simulink model "W03_P1"  (R2024b)
settings: Solver=ode4  StartTime=0  StopTime=T_final  FixedStep=h  RelTol=1e-3
undefined symbols (not defined in the file or in its folder): beta_c, mp, rp, V_c, x0
settings Model: Creator=admin  LastModifiedBy=admin
settings DataIOCC: ReturnWorkspaceOutputs=off

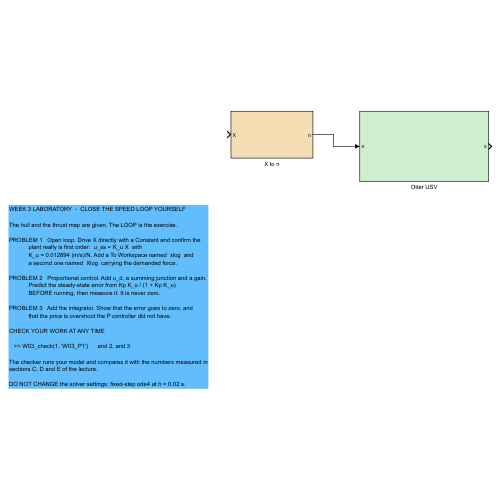
[thumbnail: Simulink's stored preview of the top-level diagram]
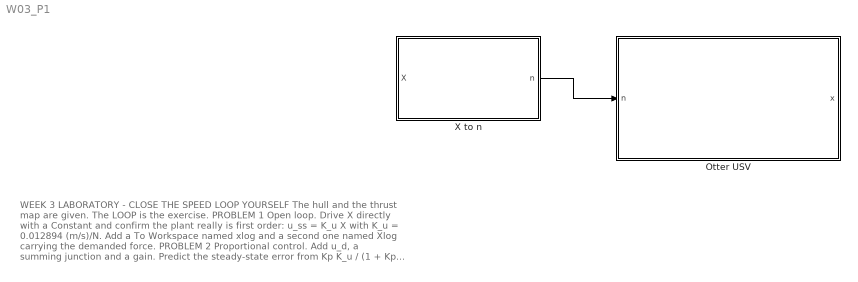
== system W03_P1 ==
  note: WEEK 3 LABORATORY  -  CLOSE THE SPEED LOOP YOURSELF
      |
      | The hull and the thrust map are given. The LOOP is the exercise.
      |
      | PROBLEM 1   Open loop. Drive X directly with a Constant and confirm the
      |             plant really is first order:  u_ss = K_u X  with
      |             K_u = 0.012894 (m/s)/N. Add a To Workspace named  xlog  and
      |             a second one named  Xlog  carrying the demanded force.
      |
      | PROBLEM 2   Proportional control. Add u_d, a summing junction and a gain.
      |             Predict the steady-state error from Kp K_u / (1 + Kp K_u)
      |             BEFORE running, then measure it. It is never zero.
      |
      | PROBLEM 3   Add the integrator. Show that the error goes to zero, and
      |             that the price is overshoot the P controller did not have.
      |
      | CHECK YOUR WORK AT ANY TIME
      |
      |    >> W03_check(1, 'W03_P1')      and 2, and 3
      |
      | The checker runs your model and compares it with the numbers measured in
      | sections C, D and E of the lecture.
      |
      | DO NOT CHANGE the solver settings: fixed-step ode4 at h = 0.02 s.
  Otter USV : Subsystem
  X to n : Subsystem
  wires:
  X to n/1(n) -> Otter USV/1(n)

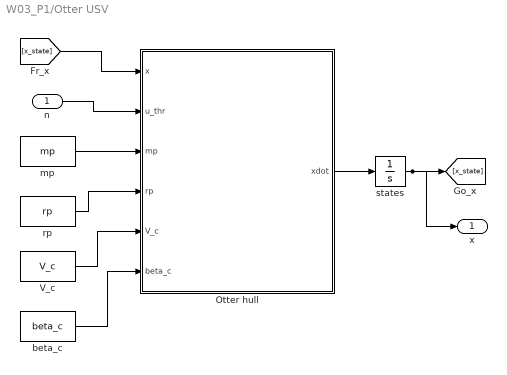
== system W03_P1/Otter USV ==
  n : Inport
  Otter hull : MATLAB Function  TreatAsAtomicUnit=on
  V_c : Constant  Value=V_c
  beta_c : Constant  Value=beta_c
  mp : Constant  Value=mp
  rp : Constant  Value=rp
  states : Integrator  InitialCondition=x0
  x : Outport
  wires:
  rp/1 -> Otter hull/4(rp)
  [x_state] -> Otter hull/1(x)
  n/1 -> Otter hull/2(u_thr)
  mp/1 -> Otter hull/3(mp)
  V_c/1 -> Otter hull/5(V_c)
  Otter hull/1(xdot) -> states/1
  beta_c/1 -> Otter hull/6(beta_c)
  states/1 -> [x_state], x/1

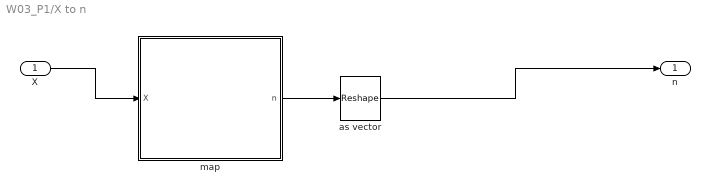
== system W03_P1/X to n ==
  X : Inport
  as vector : Reshape
  map : MATLAB Function  TreatAsAtomicUnit=on
  n : Outport
  wires:
  X/1 -> map/1(X)
  map/1(n) -> as vector/1
  as vector/1 -> n/1

== matlab function W03_P1/Otter USV/Otter hull ==
  data: x input; xdot output double size=[12 1]; u_thr input; mp input; rp input; V_c input; beta_c input
function xdot = otter_hull(x, u_thr, mp, rp, V_c, beta_c)
% Fossen's otter.m, called unchanged from Tools/MSS/VESSELS.
%
%   x       12 states, fed back from the integrator
%   u_thr   propeller shaft speeds [rad/s]
%
% otter.m is not written for code generation, so the call is extrinsic and
% xdot has to be pre-sized for Simulink to know the output width.
coder.extrinsic('otter');

xdot = zeros(12,1);
xdot = otter(x, u_thr, mp, rp, V_c, beta_c);
end

== matlab function W03_P1/X to n/map ==
  data: X input; n output double size=[2 1]
function n = map(X)
%#codegen
%MAP  Demanded surge force -> two equal shaft speeds.
%
%  Both propellers share the load, so each provides X/2, and the thrust of
%  one propeller is T = k_pos n|n| ahead, k_neg n|n| astern. Inverting that
%  and saturating at the Otter's shaft limits gives the command.
%
%  Derived in Appendix A1 section C. Provided here so that Week 3 spends
%  its hour on the controller.
k_pos = 0.02216/2;   k_neg = 0.01289/2;
n_max =  sqrt((0.5*24.4*9.81)/k_pos);
n_min = -sqrt((0.5*13.6*9.81)/k_neg);
T = X/2;
if T >= 0
    ni =  sqrt(  T  / k_pos);
else
    ni = -sqrt( -T  / k_neg);
end
ni = min(max(ni, n_min), n_max);
n  = [ni; ni];
